simulink model "mpc555_fuelsys"  (Simulink 6.0)
settings: Solver=ode3  SolverMode=SingleTasking  StartTime=0.0  StopTime=8  FixedStep=0.01  RelTol=1e-5  AbsTol=1e-6
PreLoadFcn:
  | RTWConfigurationCB('preloadfcn', bdroot);load mpc555_fuelsysdata.mat
libraries: simulink x5, mpc555_fuelsys_project x1, simulink_extras x1
CloseFcn:
  | rtwprivate ssgencode ModelCloseRequest ssdemo_pil_build
settings Model: CovMetricSettings=d  Creator=The MathWorks Inc.  LastModifiedBy=batserve  ExtModeTrigMode=oneshot  ExtModeArmWhenConnect=off  ExtModeAutoUpdateStatusClock=off  ProdHWDeviceType=Motorola PowerPC
settings DataIOCC: LimitDataPoints=off  SaveOutput=off  SaveTime=off  SignalLoggingName=sigsOut
settings OptimizationCC: BlockReduction=off  InlineParams=on  InlineInvariantSignals=off  OptimizeModelRefInitCode=on  LifeSpan=1
settings DebuggingCC: CheckExecutionContextPreStartOutputMsg=on  CheckExecutionContextRuntimeOutputMsg=on  SolverPrmCheckMsg=none  IntegerOverflowMsg=none
settings HardwareCC: ProdEndianess=BigEndian  ProdHWDeviceType=Motorola PowerPC  TargetHWDeviceType=32-bit Generic
settings ModelReferenceCC: UpdateModelReferenceTargets=IfOutOfDate
settings RTWCC: SystemTargetFile=mpc555pil.tlc  TemplateMakefile=mpc555pil_default_tmf  Description=Embedded Target for Motorola MPC555 (processor-in-the-loop)  RetainRTWFile=on  ProcessScript=mpc555pil_make_rtw_hook
settings CodeAppCC: IgnoreCustomStorageClasses=off
settings STFCustomTargetCC: TargetFcnLib=ansi_tfl_tmw.mat  GenFloatMathFcnCalls=ANSI_C  ModelReferenceCompliant=off  CombineOutputUpdateFcns=on  ERTCustomFileBanners=on  SystemTargetFile=mpc555pil.tlc
settings ERTTargetCC: TargetFcnLib=ansi_tfl_tmw.mat  GenFloatMathFcnCalls=ANSI_C  ModelReferenceCompliant=off  SupportContinuousTime=on  SupportNonInlinedSFcns=on  RootIOFormat=Individual Arguments  ERTCustomFileTemplate=example_file_process.tlc  InitialValueSource=Model
settings CustomProperty: DataType=RTWOptions_EnumType__toolbox_rtw_targets_mpc555dk_mpc555dk_mpc555pil_MPC555_OPTIMIZATION_SWITCH  Value=speed
settings EnumStrPairs: String=speed

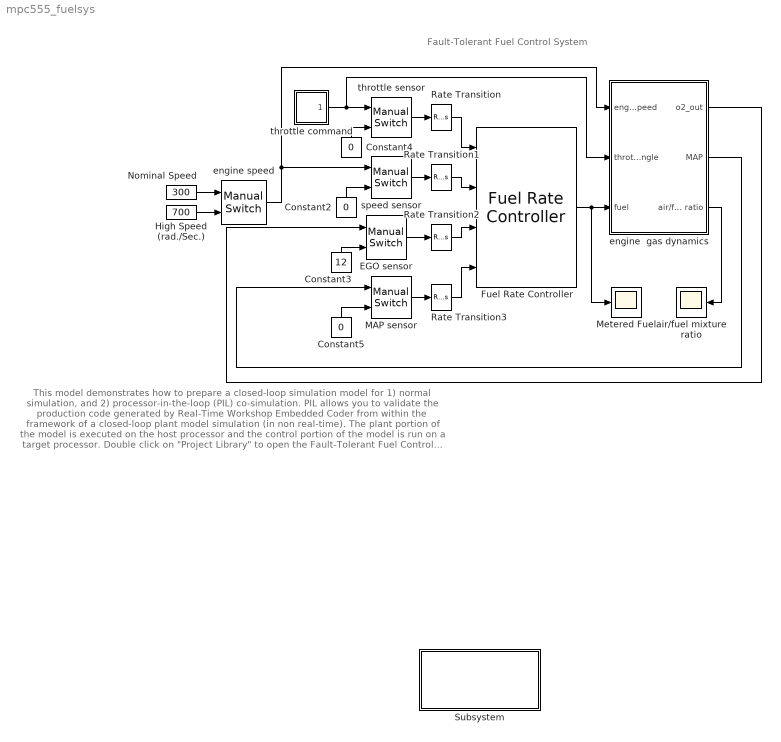
== system mpc555_fuelsys ==
  note: Fault-Tolerant Fuel Control System
  note: This model demonstrates how to prepare a closed-loop simulation model for
      | 1) normal simulation, and 2) processor-in-the-loop (PIL) co-simulation.
      |
      | PIL allows you to validate the production code generated by Real-Time Workshop
      | Embedded Coder from within the framework of a closed-loop plant model simulation
      | (in non real-time).  The plant portion of the model is executed on the host processor
      | and the control portion of the model is run on a target processor.
      |
      | Double click on "Project Library" to open the Fault-Tolerant Fuel Control System
      | Project Library. This contains the Fuel Rate Controller block used in this model, and
      | also a link to a model that deploys this control algorithm in real-time on an MPC555,
      | using target specific device driver blocks.
  Constant2 : Constant  Orientation=up  Value=0
  Constant3 : Constant  Orientation=up  Value=12
  Constant4 : Constant  Orientation=up  Value=0
  Constant5 : Constant  Orientation=up  Value=0
  EGO sensor : simulink/Signal Routing/Manual Switch  sw=1  action=0
  Fuel Rate Controller : mpc555_fuelsys_project/Fuel Rate Controller
  High Speed (rad./Sec.) : Constant  Value=700
  MAP sensor : simulink/Signal Routing/Manual Switch  sw=1  action=0
  Metered Fuel : Scope
      settings: TickLabels=on  TimeRange=8  YMin=0.75  YMax=2.25  DataFormat=Array
  Nominal Speed : Constant  Value=300
  Rate Transition{,1..3} (4 alike) : RateTransition  OutPortSampleTime=0.01
  Subsystem : Subsystem
      settings: OpenFcn=mpc555_fuelsys_project
      mask Display: disp(sprintf('Project Library'));
  air/fuel mixture ratio : Scope
      settings: TickLabels=on  TimeRange=8  YMin=11  YMax=16  DataFormat=Array
  engine speed : simulink/Signal Routing/Manual Switch  sw=1  action=0
  engine  gas dynamics : Subsystem
  speed sensor : simulink/Signal Routing/Manual Switch  sw=1  action=0
  throttle command : Subsystem  mask(Repeating table){rep_seq_t=[0 2 4], rep_seq_y=[10 20 10]}
      mask prompts: rep_seq_t "Time values:"; rep_seq_y "Output values:"
      mask help: Repeating table.
      mask init:
      | period = max(rep_seq_t);
      mask Help: Repeats cycle given in table. Time values should be monotonically increasing.
      mask Display: plot([rep_seq_t,rep_seq_t+period,rep_seq_t+2*period,rep_seq_t(1)+3*period],[rep_seq_y,rep_seq_y,rep_seq_y,rep_seq_y(1)])
  throttle sensor : simulink/Signal Routing/Manual Switch  sw=1  action=0
  wires:
  engine  gas dynamics/3(air/fuel ratio) -> air/fuel mixture ratio/1
  engine speed/1 -> speed sensor/1, engine  gas dynamics/1(engine speed)
  EGO sensor/1 -> Rate Transition2/1
  speed sensor/1 -> Rate Transition1/1
  throttle sensor/1 -> Rate Transition/1
  engine  gas dynamics/1(o2_out) -> EGO sensor/1
  Constant5/1 -> MAP sensor/2
  Constant3/1 -> EGO sensor/2
  throttle command/1(out_1) -> throttle sensor/1, engine  gas dynamics/2(throttle angle)
  Constant2/1 -> speed sensor/2
  Constant4/1 -> throttle sensor/2
  engine  gas dynamics/2(MAP) -> MAP sensor/1
  High Speed (rad./Sec.)/1 -> engine speed/2
  Nominal Speed/1 -> engine speed/1
  Fuel Rate Controller/1 -> Metered Fuel/1, engine  gas dynamics/3(fuel)
  MAP sensor/1 -> Rate Transition3/1
  Rate Transition/1 -> Fuel Rate Controller/1
  Rate Transition1/1 -> Fuel Rate Controller/2
  Rate Transition2/1 -> Fuel Rate Controller/3
  Rate Transition3/1 -> Fuel Rate Controller/4

== system mpc555_fuelsys/Subsystem ==

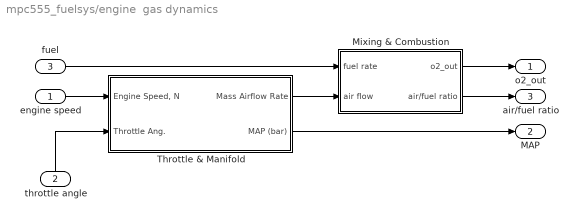
== system mpc555_fuelsys/engine  gas dynamics ==
  engine speed : Inport  Port=1  LatchInput=off
  throttle angle : Inport  Orientation=up  Port=2  LatchInput=off
  fuel : Inport  Port=3  LatchInput=off
  Mixing & Combustion : Subsystem
  Throttle & Manifold : Subsystem
  o2_out : Outport  InitialOutput=0
  MAP : Outport  Port=2  InitialOutput=0
  air/fuel ratio : Outport  Port=3  InitialOutput=0
  wires:
  Mixing & Combustion/1(o2_out) -> o2_out/1
  Throttle & Manifold/2(MAP (bar)) -> MAP/1
  Mixing & Combustion/2(air/fuel ratio) -> air/fuel ratio/1
  throttle angle/1 -> Throttle & Manifold/2(Throttle Ang.)
  engine speed/1 -> Throttle & Manifold/1("Engine Speed, N")
  fuel/1 -> Mixing & Combustion/1(fuel rate)
  Throttle & Manifold/1(Mass Airflow Rate) -> Mixing & Combustion/2(air flow)

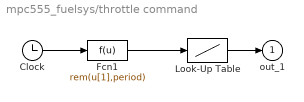
== system mpc555_fuelsys/throttle command ==
  Clock : Clock
      settings: Decimation=10
  Fcn1 : Fcn  Expr=rem(u[1],period)
  Look-Up Table : Lookup  DialogController=Simulink.DDGSource  InputValues=rep_seq_t  OutputValues=rep_seq_y  SaturateOnIntegerOverflow=on
  out_1 : Outport  InitialOutput=0
  wires:
  Look-Up Table/1 -> out_1/1
  Clock/1 -> Fcn1/1
  Fcn1/1 -> Look-Up Table/1

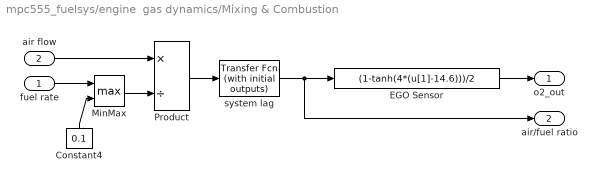
== system mpc555_fuelsys/engine  gas dynamics/Mixing & Combustion ==
  fuel rate : Inport  Port=1  LatchInput=off
  air flow : Inport  Port=2  LatchInput=off
  Constant4 : Constant  Orientation=up  Value=0.1
  EGO Sensor : Fcn  Expr=(1-tanh(4*(u[1]-14.6)))/2
  MinMax : MinMax  Function=max  Inputs=2  SaturateOnIntegerOverflow=on  InputSameDT=on
  Product : Product  Inputs=*/  SaturateOnIntegerOverflow=on  RndMeth=Zero  InputSameDT=on
  system lag : simulink_extras/Additional Linear/Transfer Fcn (with initial outputs)  N=3  D=[1 3]  Y0=1/14.6  U0=1/14.6
  o2_out : Outport  InitialOutput=0
  air/fuel ratio : Outport  Port=2  InitialOutput=0
  wires:
  air flow/1 -> Product/1
  EGO Sensor/1 -> o2_out/1
  system lag/1 -> EGO Sensor/1, air/fuel ratio/1
  Product/1 -> system lag/1
  MinMax/1 -> Product/2
  fuel rate/1 -> MinMax/1
  Constant4/1 -> MinMax/2

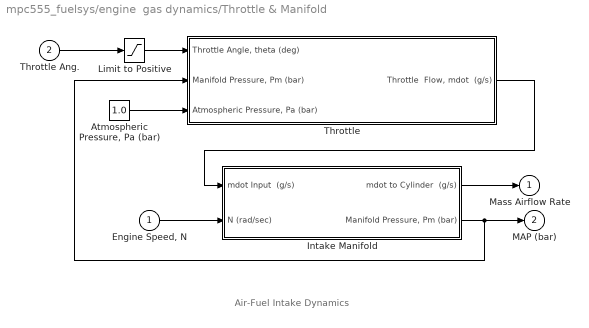
== system mpc555_fuelsys/engine  gas dynamics/Throttle & Manifold ==
  note: Air-Fuel Intake Dynamics
  "Engine Speed, N" : Inport  Port=1  LatchInput=off
  Throttle Ang. : Inport  Port=2  LatchInput=off
  "Atmospheric Pressure, Pa (bar)" : Constant  Value=1.0
  Intake Manifold : Subsystem
  Limit to Positive : Saturate  UpperLimit=inf  LowerLimit=0
  Throttle : Subsystem
  Mass Airflow Rate : Outport  InitialOutput=0
  MAP (bar) : Outport  Port=2  InitialOutput=0
  wires:
  Intake Manifold/2("Manifold Pressure, Pm (bar)") -> MAP (bar)/1, Throttle/2("Manifold Pressure, Pm (bar)")
  "Atmospheric Pressure, Pa (bar)"/1 -> Throttle/3("Atmospheric Pressure, Pa (bar) ")
  Intake Manifold/1(mdot to Cylinder  (g/s)) -> Mass Airflow Rate/1
  "Engine Speed, N"/1 -> Intake Manifold/2(N (rad/sec))
  Throttle/1("Throttle  Flow, mdot  (g/s)") -> Intake Manifold/1(mdot Input  (g/s))
  Throttle Ang./1 -> Limit to Positive/1
  Limit to Positive/1 -> Throttle/1("Throttle Angle, theta (deg)")

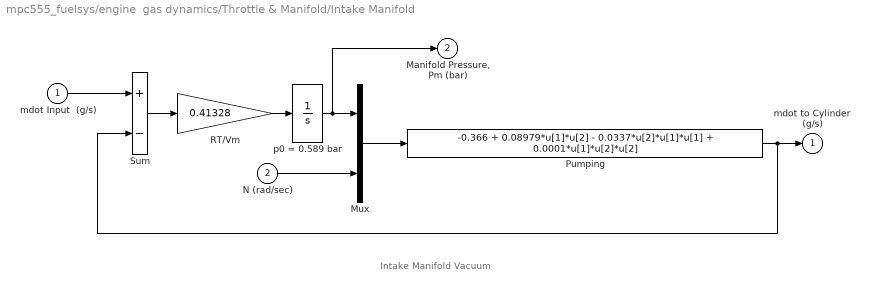
== system mpc555_fuelsys/engine  gas dynamics/Throttle & Manifold/Intake Manifold ==
  note: Intake Manifold Vacuum
  mdot Input  (g/s) : Inport  Port=1  LatchInput=off
  N (rad/sec) : Inport  Port=2  LatchInput=off
  Mux : Mux  Inputs=2
  Pumping : Fcn  Expr=-0.366 + 0.08979*u[1]*u[2] - 0.0337*u[2]*u[1]*u[1] + 0.0001*u[1]*u[2]*u[2]
  RT/Vm : Gain  Gain=0.41328  SaturateOnIntegerOverflow=on
  Sum : Sum  Inputs=+-  SaturateOnIntegerOverflow=on  InputSameDT=on
  p0 = 0.589 bar : Integrator  InitialCondition=.589
  mdot to Cylinder  (g/s) : Outport  InitialOutput=0
  "Manifold Pressure, Pm (bar)" : Outport  Port=2  InitialOutput=0
  wires:
  Pumping/1 -> mdot to Cylinder  (g/s)/1, Sum/2
  Sum/1 -> RT/Vm/1
  p0 = 0.589 bar/1 -> "Manifold Pressure, Pm (bar)"/1, Mux/1
  Mux/1 -> Pumping/1
  N (rad/sec)/1 -> Mux/2
  RT/Vm/1 -> p0 = 0.589 bar/1
  mdot Input  (g/s)/1 -> Sum/1

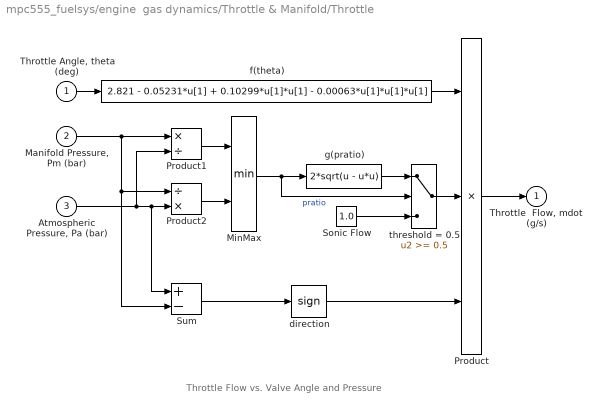
== system mpc555_fuelsys/engine  gas dynamics/Throttle & Manifold/Throttle ==
  note: Throttle Flow vs. Valve Angle and Pressure
  "Throttle Angle, theta (deg)" : Inport  Port=1  LatchInput=off
  "Manifold Pressure, Pm (bar)" : Inport  Port=2  LatchInput=off
  "Atmospheric Pressure, Pa (bar) " : Inport  Port=3  LatchInput=off
  MinMax : MinMax  Inputs=2  SaturateOnIntegerOverflow=on  InputSameDT=on
  Product : Product  Inputs=3  SaturateOnIntegerOverflow=on  RndMeth=Zero  InputSameDT=on
  Product1 : Product  Inputs=*/  SaturateOnIntegerOverflow=on  RndMeth=Zero  InputSameDT=on
  Product2 : Product  Inputs=/*  SaturateOnIntegerOverflow=on  RndMeth=Zero  InputSameDT=on
  "Sonic Flow " : Constant  Value=1.0
  Sum : Sum  Inputs=+-  SaturateOnIntegerOverflow=on  InputSameDT=on
  direction : Signum
  f(theta) : Fcn  Expr=2.821 - 0.05231*u[1] + 0.10299*u[1]*u[1] - 0.00063*u[1]*u[1]*u[1]
  g(pratio) : Fcn  Expr=2*sqrt(u - u*u)
  threshold = 0.5 : Switch  Threshold=0.5  SaturateOnIntegerOverflow=on  InputSameDT=on
  "Throttle  Flow, mdot  (g/s)" : Outport  InitialOutput=0
  wires:
  f(theta)/1 -> Product/1
  Product/1 -> "Throttle  Flow, mdot  (g/s)"/1
  "Throttle Angle, theta (deg)"/1 -> f(theta)/1
  MinMax/1 -> g(pratio)/1, threshold = 0.5/2  "pratio"
  Sum/1 -> direction/1
  direction/1 -> Product/3
  threshold = 0.5/1 -> Product/2
  "Sonic Flow "/1 -> threshold = 0.5/3
  g(pratio)/1 -> threshold = 0.5/1
  "Atmospheric Pressure, Pa (bar) "/1 -> Product1/2, Product2/2, Sum/1
  Product1/1 -> MinMax/1
  Product2/1 -> MinMax/2
  "Manifold Pressure, Pm (bar)"/1 -> Product1/1, Product2/1, Sum/2
